simulink model "RaibertControlV2"  (R2022a)
settings: Solver=ode4  StartTime=0.0  StopTime=1  FixedStep=1/1000  RelTol=1e-3  AbsTol=1e-3  EnableMultiTasking=on
undefined symbols (not defined in the file or in its folder): Carrier, N, Ring, T, X, Y, Z
libraries: sm_lib x133, nesl_utility x25, Multibody_Parts_Lib x4, fl_lib x4
(part 6 of 8)

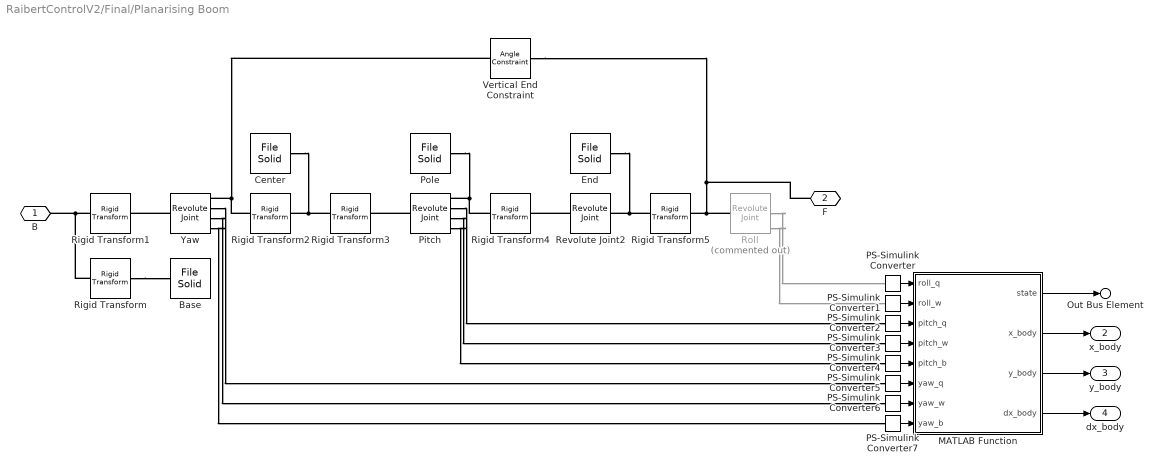
== system RaibertControlV2/Final/Planarising Boom ==
  Base : sm_lib/Body Elements/File Solid  ExtGeomFileName=meshes/boom_base.stl  UnitType=Custom  ExtGeomFileUnits=mm  StepReaderType=HEX  ExportConvexHullGeometry=off  InertiaType=Custom  Mass=16346.96  MassUnits=g  CenterOfMass=[0 10.41 0]  CenterOfMassUnits=mm  MomentsOfInertia=[161213573.39 313845541.56 161213574.63]  MomentsOfInertiaUnits=g*mm^2  ProductsOfInertia=-[32.04 0 0]  ProductsOfInertiaUnits=g*mm^2  BasedOnType=Density  Density=1000  DensityUnits=kg/m^3  DoExposeReferenceFrame=on  SerializedFrames=<Frames/>  GraphicType=FromGeometry  MarkerShape=Sphere  MarkerSize=10  GraphicVisPropType=AdvancedVisualProperties  GraphicDiffuseColor=Boom.Base.color  GraphicSpecularColor=[0.5 0.5 0.5 1.0]  GraphicAmbientColor=[0.15 0.15 0.15 1.0]  GraphicEmissiveColor=[0.0 0.0 0.0 1.0]  GraphicShininess=75  GraphicOpacity=1.0
  Center : sm_lib/Body Elements/File Solid  ExtGeomFileName=meshes/boom_center.stl  UnitType=Custom  ExtGeomFileUnits=mm  StepReaderType=HEX  ExportConvexHullGeometry=off  InertiaType=Custom  Mass=714.59  MassUnits=g  CenterOfMass=[9.30 7.66 -1.81]  CenterOfMassUnits=mm  MomentsOfInertia=[927484.76 701141.66 1377594.42]  MomentsOfInertiaUnits=g*mm^2  ProductsOfInertia=-[9906.49 -12376.64 180221.56]  ProductsOfInertiaUnits=g*mm^2  BasedOnType=Density  Density=1000  DensityUnits=kg/m^3  DoExposeReferenceFrame=on  SerializedFrames=<Frames/>  GraphicType=FromGeometry  MarkerShape=Sphere  MarkerSize=10  GraphicVisPropType=AdvancedVisualProperties  GraphicDiffuseColor=Boom.Center.color  GraphicSpecularColor=[0.5 0.5 0.5 1.0]  GraphicAmbientColor=[0.15 0.15 0.15 1.0]  GraphicEmissiveColor=[0.0 0.0 0.0 1.0]  GraphicShininess=75  GraphicOpacity=1.0
  End : sm_lib/Body Elements/File Solid  ExtGeomFileName=meshes/boom_end.stl  UnitType=Custom  ExtGeomFileUnits=mm  StepReaderType=HEX  ExportConvexHullGeometry=off  InertiaType=Custom  Mass=228  MassUnits=g  CenterOfMass=[14.63 3.02 0]  CenterOfMassUnits=mm  MomentsOfInertia=[116760.20 135814.15 68848.95]  MomentsOfInertiaUnits=g*mm^2  ProductsOfInertia=-[0 0 -1218.21]  ProductsOfInertiaUnits=g*mm^2  BasedOnType=Density  Density=1000  DensityUnits=kg/m^3  DoExposeReferenceFrame=on  SerializedFrames=<Frames/>  GraphicType=FromGeometry  MarkerShape=Sphere  MarkerSize=10  GraphicVisPropType=AdvancedVisualProperties  GraphicDiffuseColor=Boom.End.color  GraphicSpecularColor=[0.5 0.5 0.5 1.0]  GraphicAmbientColor=[0.15 0.15 0.15 1.0]  GraphicEmissiveColor=[0.0 0.0 0.0 1.0]  GraphicShininess=75  GraphicOpacity=1.0
  MATLAB Function : MATLAB Function  TreatAsAtomicUnit=on
  PS-Simulink Converter{,1..7} (8 alike) : nesl_utility/PS-Simulink Converter  PhysicalDomain=network_engine_domain  SubClassName=ps_output  LeftPortType=input  RightPortType=output  PseudoPeriodic=off  Frequencies=[]  VectorFormat=inherit  Unit=inherit  AffineConversion=off
      settings: SourceProductBaseCode=SS,PW,VE
  Pitch : sm_lib/Joints/Revolute Joint  JointMode=Normal  SenseConstraintForce=off  SenseConstraintForceX=off  SenseConstraintForceY=off  SenseConstraintForceZ=off  SenseConstraintTorque=off  SenseConstraintTorqueX=off  SenseConstraintTorqueY=off  SenseConstraintTorqueZ=off  SenseTotalForce=off  SenseTotalForceX=off  SenseTotalForceY=off  SenseTotalForceZ=off  SenseTotalTorque=off  SenseTotalTorqueX=off  SenseTotalTorqueY=off  SenseTotalTorqueZ=off  CompositeWrenchDir=FollowerOnBase  CompositeWrenchFrame=BaseFrame  EquilibriumPosition=0  EquilibriumPositionUnits=deg  SpringStiffness=0  SpringStiffnessUnits=N*m/deg  DampingCoefficient=0  DampingCoefficientUnits=N*m/(deg/s)  TorqueActuationMode=NoTorque  MotionActuationMode=ComputedMotion  SensePosition=on  SenseVelocity=on  SenseAcceleration=on  SenseTorqueForce=off  SenseLowerLimitTorqueForce=off  SenseUpperLimitTorqueForce=off  LowerLimitSpecify=off  LowerLimitBound=-90  LowerLimitBoundUnits=deg  LowerLimitStiffness=1e4  LowerLimitStiffnessUnits=N*m/deg  LowerLimitDamping=10  LowerLimitDampingUnits=N*m/(deg/s)  LowerLimitTransitionRegionWidth=0.1  LowerLimitTransitionRegionWidthUnits=deg  UpperLimitSpecify=off  UpperLimitBound=90  UpperLimitBoundUnits=deg  UpperLimitStiffness=1e4  UpperLimitStiffnessUnits=N*m/deg  UpperLimitDamping=10  UpperLimitDampingUnits=N*m/(deg/s)  UpperLimitTransitionRegionWidth=0.1  UpperLimitTransitionRegionWidthUnits=deg  PositionTargetSpecify=on  PositionTargetPriority=High  PositionTargetValue=25  PositionTargetValueUnits=deg  VelocityTargetSpecify=off  VelocityTargetPriority=High  VelocityTargetValue=10  VelocityTargetValueUnits=deg/s
  Pole : sm_lib/Body Elements/File Solid  ExtGeomFileName=meshes/boom_pole.stl  UnitType=Custom  ExtGeomFileUnits=mm  StepReaderType=HEX  ExportConvexHullGeometry=off  InertiaType=Custom  Mass=2470.66  MassUnits=g  CenterOfMass=[1149.01 0 0.46]  CenterOfMassUnits=mm  MomentsOfInertia=[1403119.37 1561987235.33 1561886539.18]  MomentsOfInertiaUnits=g*mm^2  ProductsOfInertia=-[-8.91 -1292286.42 224.67]  ProductsOfInertiaUnits=g*mm^2  BasedOnType=Density  Density=1000  DensityUnits=kg/m^3  DoExposeReferenceFrame=on  SerializedFrames=<Frames/>  GraphicType=FromGeometry  MarkerShape=Sphere  MarkerSize=10  GraphicVisPropType=AdvancedVisualProperties  GraphicDiffuseColor=Boom.Pole.color  GraphicSpecularColor=[0.5 0.5 0.5 1.0]  GraphicAmbientColor=[0.15 0.15 0.15 1.0]  GraphicEmissiveColor=[0.0 0.0 0.0 1.0]  GraphicShininess=75  GraphicOpacity=1.0
  Revolute Joint2 : sm_lib/Joints/Revolute Joint  JointMode=Normal  SenseConstraintForce=off  SenseConstraintForceX=off  SenseConstraintForceY=off  SenseConstraintForceZ=off  SenseConstraintTorque=off  SenseConstraintTorqueX=off  SenseConstraintTorqueY=off  SenseConstraintTorqueZ=off  SenseTotalForce=off  SenseTotalForceX=off  SenseTotalForceY=off  SenseTotalForceZ=off  SenseTotalTorque=off  SenseTotalTorqueX=off  SenseTotalTorqueY=off  SenseTotalTorqueZ=off  CompositeWrenchDir=FollowerOnBase  CompositeWrenchFrame=BaseFrame  EquilibriumPosition=0  EquilibriumPositionUnits=deg  SpringStiffness=0  SpringStiffnessUnits=N*m/deg  DampingCoefficient=0  DampingCoefficientUnits=N*m/(deg/s)  TorqueActuationMode=NoTorque  MotionActuationMode=ComputedMotion  SensePosition=off  SenseVelocity=off  SenseAcceleration=off  SenseTorqueForce=off  SenseLowerLimitTorqueForce=off  SenseUpperLimitTorqueForce=off  LowerLimitSpecify=off  LowerLimitBound=-90  LowerLimitBoundUnits=deg  LowerLimitStiffness=1e4  LowerLimitStiffnessUnits=N*m/deg  LowerLimitDamping=10  LowerLimitDampingUnits=N*m/(deg/s)  LowerLimitTransitionRegionWidth=0.1  LowerLimitTransitionRegionWidthUnits=deg  UpperLimitSpecify=off  UpperLimitBound=90  UpperLimitBoundUnits=deg  UpperLimitStiffness=1e4  UpperLimitStiffnessUnits=N*m/deg  UpperLimitDamping=10  UpperLimitDampingUnits=N*m/(deg/s)  UpperLimitTransitionRegionWidth=0.1  UpperLimitTransitionRegionWidthUnits=deg  PositionTargetSpecify=off  PositionTargetPriority=High  PositionTargetValue=0  PositionTargetValueUnits=deg  VelocityTargetSpecify=off  VelocityTargetPriority=High  VelocityTargetValue=0  VelocityTargetValueUnits=deg/s
  Rigid Transform : sm_lib/Frames and Transforms/Rigid Transform  TranslationMethod=None  TranslationStandardOffset=0  TranslationLengthUnit=m  TranslationStandardAxis=+Z  TranslationCartesianOffset=[0 0 0]  TranslationROffset=0  TranslationROffsetUnits=m  TranslationZOffset=0  TranslationZOffsetUnits=m  TranslationThetaOffset=0  TranslationThetaOffsetUnits=deg  RotationMethod=AlignedAxes  RotationAngleUnits=deg  RotationStandardAxis=+Z  RotationAngle=0.0  RotationArbitraryAxis=[0 0 1]  FollAlignAxisA=+Y  BaseAlignAxisA=+Z  FollAlignAxisB=+X  BaseAlignAxisB=+X  RotationSequenceAxes=FollowerAxes  RotationSequence=XYX  RotationSequenceAngles=[0 0 0]  RotationSequenceAnglesUnits=deg  RotationMatrix=[1 0 0; 0 1 0; 0 0 1]
  Rigid Transform1 : sm_lib/Frames and Transforms/Rigid Transform  TranslationMethod=StandardAxis  TranslationStandardOffset=101  TranslationLengthUnit=mm  TranslationStandardAxis=+Z  TranslationCartesianOffset=[0 0 101]  TranslationROffset=0  TranslationROffsetUnits=m  TranslationZOffset=0  TranslationZOffsetUnits=m  TranslationThetaOffset=0  TranslationThetaOffsetUnits=deg  RotationMethod=None  RotationAngleUnits=deg  RotationStandardAxis=+Z  RotationAngle=0.0  RotationArbitraryAxis=[0 0 1]  FollAlignAxisA=+Y  BaseAlignAxisA=+Z  FollAlignAxisB=+X  BaseAlignAxisB=+X  RotationSequenceAxes=FollowerAxes  RotationSequence=XYX  RotationSequenceAngles=[0 0 0]  RotationSequenceAnglesUnits=deg  RotationMatrix=[1 0 0; 0 1 0; 0 0 1]
  Rigid Transform2 : sm_lib/Frames and Transforms/Rigid Transform  TranslationMethod=None  TranslationStandardOffset=0  TranslationLengthUnit=mm  TranslationStandardAxis=+Z  TranslationCartesianOffset=[0 0 101]  TranslationROffset=0  TranslationROffsetUnits=m  TranslationZOffset=0  TranslationZOffsetUnits=m  TranslationThetaOffset=0  TranslationThetaOffsetUnits=deg  RotationMethod=AlignedAxes  RotationAngleUnits=deg  RotationStandardAxis=+Z  RotationAngle=0.0  RotationArbitraryAxis=[0 0 1]  FollAlignAxisA=+Y  BaseAlignAxisA=+Z  FollAlignAxisB=+X  BaseAlignAxisB=-X  RotationSequenceAxes=FollowerAxes  RotationSequence=XYX  RotationSequenceAngles=[0 0 0]  RotationSequenceAnglesUnits=deg  RotationMatrix=[1 0 0; 0 1 0; 0 0 1]
  Rigid Transform3 : sm_lib/Frames and Transforms/Rigid Transform  TranslationMethod=StandardAxis  TranslationStandardOffset=40  TranslationLengthUnit=mm  TranslationStandardAxis=-X  TranslationCartesianOffset=[-40 0 0]  TranslationROffset=0  TranslationROffsetUnits=m  TranslationZOffset=0  TranslationZOffsetUnits=m  TranslationThetaOffset=0  TranslationThetaOffsetUnits=deg  RotationMethod=AlignedAxes  RotationAngleUnits=deg  RotationStandardAxis=+Z  RotationAngle=0.0  RotationArbitraryAxis=[0 0 1]  FollAlignAxisA=+Y  BaseAlignAxisA=+Y  FollAlignAxisB=+X  BaseAlignAxisB=-X  RotationSequenceAxes=FollowerAxes  RotationSequence=XYX  RotationSequenceAngles=[0 0 0]  RotationSequenceAnglesUnits=deg  RotationMatrix=[1 0 0; 0 1 0; 0 0 1]
  Rigid Transform4 : sm_lib/Frames and Transforms/Rigid Transform  TranslationMethod=StandardAxis  TranslationStandardOffset=2493  TranslationLengthUnit=mm  TranslationStandardAxis=+X  TranslationCartesianOffset=[2493 0 0]  TranslationROffset=0  TranslationROffsetUnits=m  TranslationZOffset=0  TranslationZOffsetUnits=m  TranslationThetaOffset=0  TranslationThetaOffsetUnits=deg  RotationMethod=None  RotationAngleUnits=deg  RotationStandardAxis=+Z  RotationAngle=0.0  RotationArbitraryAxis=[0 0 1]  FollAlignAxisA=+Y  BaseAlignAxisA=+Y  FollAlignAxisB=+X  BaseAlignAxisB=-X  RotationSequenceAxes=FollowerAxes  RotationSequence=XYX  RotationSequenceAngles=[0 0 0]  RotationSequenceAnglesUnits=deg  RotationMatrix=[1 0 0; 0 1 0; 0 0 1]
  Rigid Transform5 : sm_lib/Frames and Transforms/Rigid Transform  TranslationMethod=StandardAxis  TranslationStandardOffset=83.5*0.62  TranslationLengthUnit=mm  TranslationStandardAxis=+X  TranslationCartesianOffset=[2493 0 0]  TranslationROffset=0  TranslationROffsetUnits=m  TranslationZOffset=0  TranslationZOffsetUnits=m  TranslationThetaOffset=0  TranslationThetaOffsetUnits=deg  RotationMethod=AlignedAxes  RotationAngleUnits=deg  RotationStandardAxis=+Z  RotationAngle=0.0  RotationArbitraryAxis=[0 0 1]  FollAlignAxisA=+Y  BaseAlignAxisA=+Y  FollAlignAxisB=+Z  BaseAlignAxisB=+X  RotationSequenceAxes=FollowerAxes  RotationSequence=XYX  RotationSequenceAngles=[0 0 0]  RotationSequenceAnglesUnits=deg  RotationMatrix=[1 0 0; 0 1 0; 0 0 1]
  Roll : sm_lib/Joints/Revolute Joint  Commented=on  JointMode=Normal  SenseConstraintForce=off  SenseConstraintForceX=off  SenseConstraintForceY=off  SenseConstraintForceZ=off  SenseConstraintTorque=off  SenseConstraintTorqueX=off  SenseConstraintTorqueY=off  SenseConstraintTorqueZ=off  SenseTotalForce=off  SenseTotalForceX=off  SenseTotalForceY=off  SenseTotalForceZ=off  SenseTotalTorque=off  SenseTotalTorqueX=off  SenseTotalTorqueY=off  SenseTotalTorqueZ=off  CompositeWrenchDir=FollowerOnBase  CompositeWrenchFrame=BaseFrame  EquilibriumPosition=0  EquilibriumPositionUnits=deg  SpringStiffness=0  SpringStiffnessUnits=N*m/deg  DampingCoefficient=0  DampingCoefficientUnits=N*m/(deg/s)  TorqueActuationMode=NoTorque  MotionActuationMode=ComputedMotion  SensePosition=on  SenseVelocity=on  SenseAcceleration=off  SenseTorqueForce=off  SenseLowerLimitTorqueForce=off  SenseUpperLimitTorqueForce=off  LowerLimitSpecify=off  LowerLimitBound=-90  LowerLimitBoundUnits=deg  LowerLimitStiffness=1e4  LowerLimitStiffnessUnits=N*m/deg  LowerLimitDamping=10  LowerLimitDampingUnits=N*m/(deg/s)  LowerLimitTransitionRegionWidth=0.1  LowerLimitTransitionRegionWidthUnits=deg  UpperLimitSpecify=off  UpperLimitBound=90  UpperLimitBoundUnits=deg  UpperLimitStiffness=1e4  UpperLimitStiffnessUnits=N*m/deg  UpperLimitDamping=10  UpperLimitDampingUnits=N*m/(deg/s)  UpperLimitTransitionRegionWidth=0.1  UpperLimitTransitionRegionWidthUnits=deg  PositionTargetSpecify=off  PositionTargetPriority=High  PositionTargetValue=0  PositionTargetValueUnits=deg  VelocityTargetSpecify=off  VelocityTargetPriority=High  VelocityTargetValue=10  VelocityTargetValueUnits=deg/s
  Vertical End Constraint : sm_lib/Constraints/Angle Constraint  ConstraintType=General  Angle=90  AngleUnits=deg  SenseSignedTorqueMagnitude=off  SenseTorque=off  SenseForce=off  WrenchDir=FollowerOnBase  WrenchFrame=BaseFrame
      settings: SourceProductBaseCode=MS
  Yaw : sm_lib/Joints/Revolute Joint  JointMode=Normal  SenseConstraintForce=off  SenseConstraintForceX=off  SenseConstraintForceY=off  SenseConstraintForceZ=off  SenseConstraintTorque=off  SenseConstraintTorqueX=off  SenseConstraintTorqueY=off  SenseConstraintTorqueZ=off  SenseTotalForce=off  SenseTotalForceX=off  SenseTotalForceY=off  SenseTotalForceZ=off  SenseTotalTorque=off  SenseTotalTorqueX=off  SenseTotalTorqueY=off  SenseTotalTorqueZ=off  CompositeWrenchDir=FollowerOnBase  CompositeWrenchFrame=BaseFrame  EquilibriumPosition=0  EquilibriumPositionUnits=deg  SpringStiffness=0  SpringStiffnessUnits=N*m/deg  DampingCoefficient=0  DampingCoefficientUnits=N*m/(deg/s)  TorqueActuationMode=NoTorque  MotionActuationMode=ComputedMotion  SensePosition=on  SenseVelocity=on  SenseAcceleration=on  SenseTorqueForce=off  SenseLowerLimitTorqueForce=off  SenseUpperLimitTorqueForce=off  LowerLimitSpecify=off  LowerLimitBound=-90  LowerLimitBoundUnits=deg  LowerLimitStiffness=1e4  LowerLimitStiffnessUnits=N*m/deg  LowerLimitDamping=10  LowerLimitDampingUnits=N*m/(deg/s)  LowerLimitTransitionRegionWidth=0.1  LowerLimitTransitionRegionWidthUnits=deg  UpperLimitSpecify=off  UpperLimitBound=90  UpperLimitBoundUnits=deg  UpperLimitStiffness=1e4  UpperLimitStiffnessUnits=N*m/deg  UpperLimitDamping=10  UpperLimitDampingUnits=N*m/(deg/s)  UpperLimitTransitionRegionWidth=0.1  UpperLimitTransitionRegionWidthUnits=deg  PositionTargetSpecify=off  PositionTargetPriority=High  PositionTargetValue=0  PositionTargetValueUnits=deg  VelocityTargetSpecify=off  VelocityTargetPriority=High  VelocityTargetValue=10  VelocityTargetValueUnits=deg/s
  B : PMIOPort  Side=Left
  F : PMIOPort  Port=2  Side=Right
  Out Bus Element : Outport  PortName=state
  x_body : Outport  Port=2
  y_body : Outport  Port=3
  dx_body : Outport  Port=4
  wires:
  PS-Simulink Converter/1 -> MATLAB Function/1(roll_q)
  PS-Simulink Converter1/1 -> MATLAB Function/2(roll_w)
  PS-Simulink Converter2/1 -> MATLAB Function/3(pitch_q)
  PS-Simulink Converter3/1 -> MATLAB Function/4(pitch_w)
  PS-Simulink Converter4/1 -> MATLAB Function/5(pitch_b)
  PS-Simulink Converter5/1 -> MATLAB Function/6(yaw_q)
  PS-Simulink Converter6/1 -> MATLAB Function/7(yaw_w)
  PS-Simulink Converter7/1 -> MATLAB Function/8(yaw_b)
  MATLAB Function/1(state) -> Out Bus Element/1
  MATLAB Function/3(y_body) -> y_body/1
  MATLAB Function/2(x_body) -> x_body/1
  MATLAB Function/4(dx_body) -> dx_body/1
  connections:
  Revolute Joint2/LConn1 -- Rigid Transform4/RConn1
  Pole/RConn1 -- Rigid Transform4/LConn1 -- Pitch/RConn1
  Center/RConn1 -- Rigid Transform3/LConn1 -- Rigid Transform2/RConn1
  Rigid Transform2/LConn1 -- Vertical End Constraint/LConn1 -- Yaw/RConn1
  End/RConn1 -- Rigid Transform5/LConn1 -- Revolute Joint2/RConn1
  Vertical End Constraint/RConn1 -- Roll/LConn1 -- Rigid Transform5/RConn1 -- F/RConn1
  Rigid Transform/RConn1 -- Base/RConn1
  Pitch/LConn1 -- Rigid Transform3/RConn1
  Rigid Transform/LConn1 -- B/RConn1 -- Rigid Transform1/LConn1
  Yaw/LConn1 -- Rigid Transform1/RConn1
  Roll/RConn2 -- PS-Simulink Converter/LConn1
  Roll/RConn3 -- PS-Simulink Converter1/LConn1
  Pitch/RConn2 -- PS-Simulink Converter2/LConn1
  Pitch/RConn3 -- PS-Simulink Converter3/LConn1
  Pitch/RConn4 -- PS-Simulink Converter4/LConn1
  Yaw/RConn2 -- PS-Simulink Converter5/LConn1
  Yaw/RConn3 -- PS-Simulink Converter6/LConn1
  Yaw/RConn4 -- PS-Simulink Converter7/LConn1

== matlab function RaibertControlV2/Final/AK90-M4/MATLAB Function ==
  data: tff_cmd input; q_cmd input; w_cmd input; Kp_cmd input; Kd_cmd input; q input; t output; w input
function t = PD(tff_cmd,q_cmd,w_cmd,Kp_cmd,Kd_cmd,q,w)
t = Kp_cmd*(q_cmd - q) + Kd_cmd*(w_cmd - w) + tff_cmd;

%function t = PD(cmd,q,w)
%t = cmd.Kp*(cmd.q - q) + cmd.Kd*(cmd.w - w) + cmd.tff;

== matlab function RaibertControlV2/Final/AK90-M3/MATLAB Function ==
  data: tff_cmd input; q_cmd input; w_cmd input; Kp_cmd input; Kd_cmd input; q input; t output; w input
function t = PD(tff_cmd,q_cmd,w_cmd,Kp_cmd,Kd_cmd,q,w)
t = Kp_cmd*(q_cmd - q) + Kd_cmd*(w_cmd - w) + tff_cmd;

%function t = PD(cmd,q,w)
%t = cmd.Kp*(cmd.q - q) + cmd.Kd*(cmd.w - w) + cmd.tff;

== matlab function RaibertControlV2/Final/Impedance Control/MATLAB Function3 ==
  data: state input; contact_offset input; stance_timer input; state output; contact_offset output; stance_timer output; t input; x_des input; x_body input; y_body input; dx_body input; foot_height output; r output; phi output; tau1 output; tau2 output; F_push input; theta1 input; theta2 input; r input; phi input; r_ref input; phi_ref input; dr input; dphi input; JT11 input; JT12 input; JT21 input; JT22 input
function [state,contact_offset,stance_timer,foot_height,r,phi,tau1,tau2]  = Controller(state,contact_offset,stance_timer,t,x_des,x_body,y_body,dx_body,F_push,theta1,theta2,r,phi,r_ref,phi_ref,dr,dphi,JT11,JT12,JT21,JT22)
%%
%     JT = [JT11,JT12;JT21,JT22];
% 
%     y_foot = r*cos(phi); % +ve value
%     % y_body --> +ve
%     % dx_body
%     
%     % constants
%     phi_neutral = phi_ref;
%     r0 = r_ref; % 0.38 0.33
%     r_min = 0.3; % 0.30 0.25
%     dt = 0.002;
%     
%     persistent state
%     persistent phi0
%     persistent contact_offset
%     persistent foot_contact
%     persistent Ts
%     persistent stance_timer
%     
%     if isempty(state)
%         state = State.Flight; %Loading
%     end
%     if isempty(phi0)
%         phi0 = phi_neutral;
%     end
%     if isempty(contact_offset)
%         contact_offset = 0;
%     end
%     if isempty(Ts)
%         Ts = 0.23; % 0.175
%     end
%     if isempty(stance_timer)
%         stance_timer = 0;
%     end
%     
%     % calculate foot contact
%     foot_height = y_body - y_foot- contact_offset; % This gets the foot height distance %- contact_offset;
%     if (foot_height > 0.005)
%         foot_contact = false;
%     else
%         foot_contact = true;
%     end
%     
%     % update stance duration
%     if foot_contact
%         stance_timer = stance_timer + dt;
%     end
%     
%     % state transitions
%     switch(state)
%     
%         case State.Flight
%             if foot_contact
%                 state = State.Loading;
%             end
%     
%         case State.Loading
%             if (dr < 0)
%                 state = State.Compression;
%             end
%     
%         case State.Compression
%             % leg velocity isn't always exactly zero
%             if ((-0.1 < dr && dr < 0.1) && (r < r_min))
%                 state = State.Thrust;
%                 contact_offset = y_body - y_foot; % update foot contact offset
%             end
%         case State.Thrust
%             if (r > r0)
%                 state = State.Unloading;
%             end
%         case State.Unloading
%             if not(foot_contact)
%                 state = State.Flight;
%                 Ts = min(stance_timer, 0.28); % record stance time
%                 stance_timer = 0; % reset stance timer
%             end
%     
%     end
%     
%     % radial thrust control
%     switch(state)
%         case State.Thrust
%             F_thrust = F_push;
%         otherwise
%             F_thrust = 0;
%     end
%     
%     % tau phi control
%     switch(state)
%         case State.Flight
%             % adjust foot placement based on horizontal velocity
%             dx_des = -min(max(1.0*(x_body - x_des), -0.5), 0.5);
%             x_foot = 0.5*dx_body*0.18 + 0.02*(dx_body - dx_des);
%             phi0 = phi_neutral + asin(x_foot / r0);
%             tau = 10*(phi0 - phi) + 1*(0 - dphi); % position foot
%         otherwise
%             tau = 0;
%     end
%     
%     
%     % permanent radial spring damper
%     Fr = 300*(r0 - r) + 15*(0 - dr) + F_thrust;
%     
%     % transform into joint torques
%     B = JT * [Fr; tau];
%     tau1 = B(1);
%     tau2 = B(2);
%     
%     %ctrl_state = state;
%%
    JT = [JT11,JT12;JT21,JT22];

    y_foot = r*cos(phi); % +ve value
    % y_body --> +ve
    % dx_body
    
    % constants
    phi_neutral = phi_ref;
    r0 = r_ref; % 0.38 0.33
    r_min = 0.33; % 0.30 0.25
    dt = 0.002;
    

    %States (1 = Flight, 2 = Loading, 3 = Compression, 4 = Thrust, 5 = Unloading)

    if t == 0
        state = 1; 
        phi0 = phi_neutral;
        contact_offset = 0;
        Ts = 0.23; % 0.175
        stance_timer = 0;
        tau1_add = 0;
        tau2_add = 0;
    end
    
    % calculate foot contact
    foot_height = y_body - y_foot %- contact_offset; % This gets the foot height distance %- contact_offset;
    if (foot_height > 0.05)
        foot_contact = false;
    else
        foot_contact = true;
    end
    
    % update stance duration
    if foot_contact
        stance_timer = stance_timer + dt;
    end
    
   % (1 = Flight, 2 = Loading, 3 = Compression, 4 = Thrust, 5 = Unloading)
    % state transitions
    if state == 1
        if foot_contact
            state = 2;
        end
    end

    if state == 2
        if (dr < 0)
            state = 3;
        end
    end

    if state == 3
        % leg velocity isn't always exactly zero
        if ((-0.2 < dr && dr < 0.2) && (r < r_min))
            state = 4;
            contact_offset = y_body - y_foot; % update foot contact offset
        end
    end
   
    if state == 4
        if (r > r0)
            state = 5;
        end
    end

    if state == 5
        if not(foot_contact)
            state = 1;
            Ts = min(stance_timer, 0.28); % record stance time
            stance_timer = 0; % reset stance timer
        end
    end
    
    
    
    if state == 4
        F_thrust = F_push;
    else
        F_thrust = 0;
    end
    
    % tau phi control

    if state == 1
        %function [tau1_add,tau2_add,knee_distance,flag] = PUSH(t,theta1,theta2)
        % End simulation if knees are too close 
        L1 = 17.5/100;
        L2 = 17.5/100;
        L5 = 12/100;
        q1 =  pi/2 - theta1; 
        q2 =  pi/2 - theta2;
        B1 = [-0.5*L5 - L1*cos(q1) ; L1*sin(q1)];
        B2 = [0.5*L5 + L2*cos(pi-q2) ; L2*sin(pi-q2)];
        knee_distance = abs(B1(1) - B2(1));
        if knee_distance<=0.08
            
            
            tau1_add = 100*0;
            tau2_add = -100*0;
            tau = 0;
        else 
            tau1_add = 0;
            tau2_add = 0;
            % adjust foot placement based on horizontal velocity
            dx_des = -min(max(1.0*(x_body - x_des), -0.5), 0.5);
            x_foot = 0.5*dx_body*0.18 + 0.02*(dx_body - dx_des);
            phi0 = phi_neutral + asin(x_foot / r0);
            tau = 10*(phi0 - phi) + 1*(0 - dphi); % position foot
        end
    else
        tau1_add = 0;
        tau2_add = 0;
        tau = 0;
    end
    
    
    % permanent radial spring damper
    Fr = 500*(r0 - r) + 25*(0 - dr) + F_thrust;
    t
    state
    foot_contact

    % transform into joint torques
    B = JT * [Fr; tau];
    tau1 = B(1) + tau1_add;
    tau2 = B(2) + tau2_add;
    
    %ctrl_state = state;
end

== matlab function RaibertControlV2/Final/Impedance Control1/MATLAB Function1 ==
  data: x_des input; foot_height output; x_body input; y_body input; dx_body input; pos1 input; vel1 input; pos2 input; vel2 input; ctrl_state output; r output; phi output; tau1 output; tau2 output
function [foot_height,ctrl_state,r,phi,tau1,tau2] = raibert_controller(x_des,x_body,y_body,dx_body,pos1,vel1,pos2,vel2) %#codegen
% calculate kinematics
[theta1,omega1,theta2,omega2] = motor2hip(pos1,vel1,pos2,vel2);
[r,phi] = fwd_polar(theta1,theta2);
[~,y_foot] = fwd_cartesian(theta1,theta2);
A = J_polar(theta1,theta2) * [omega1; omega2];
dr = A(1);
dphi = A(2);

y_foot = r*cos(phi); % +ve value
% y_body --> +ve
% dx_body

% constants
phi_neutral = 0.0;
r0 = 0.38; % 0.38 0.33
r_min = 0.3; % 0.30 0.25
dt = 0.002;

persistent state
persistent phi0
persistent contact_offset
persistent foot_contact
persistent Ts
persistent stance_timer

if isempty(state)
    state = State.Flight; %Loading
end
if isempty(phi0)
    phi0 = phi_neutral;
end
if isempty(contact_offset)
    contact_offset = 0;
end
if isempty(Ts)
    Ts = 0.23; % 0.175
end
if isempty(stance_timer)
    stance_timer = 0;
end

% calculate foot contact
foot_height = y_body - y_foot % This gets the foot height distance %- contact_offset;
if (foot_height > 0.005)
    foot_contact = false;
else
    foot_contact = true;
end

% update stance duration
if foot_contact
    stance_timer = stance_timer + dt;
end

% state transitions
switch(state)

    case State.Flight
        if foot_contact
            state = State.Loading;
        end

    case State.Loading
        if (dr < 0)
            state = State.Compression;
        end

    case State.Compression
        % leg velocity isn't always exactly zero
        if ((-0.1 < dr && dr < 0.1) && (r < r_min))
            state = State.Thrust;
            contact_offset = y_body - y_foot; % update foot contact offset
        end
    case State.Thrust
        if (r > r0)
            state = State.Unloading;
        end
    case State.Unloading
        if not(foot_contact)
            state = State.Flight;
            Ts = min(stance_timer, 0.28); % record stance time
            stance_timer = 0; % reset stance timer
        end

end

% radial thrust control
switch(state)
    case State.Thrust
        F_thrust = 50;
    otherwise
        F_thrust = 0;
end

% tau phi control
switch(state)
    case State.Flight
        % adjust foot placement based on horizontal velocity
        dx_des = -min(max(1.0*(x_body - x_des), -0.5), 0.5);
        x_foot = 0.5*dx_body*0.18 + 0.02*(dx_body - dx_des);
        phi0 = phi_neutral + asin(x_foot / r0);
        tau = 10*(phi0 - phi) + 1*(0 - dphi); % position foot
    otherwise
        tau = 0;
end


% permanent radial spring damper
Fr = 300*(r0 - r) + 15*(0 - dr) + F_thrust;

% transform into joint torques
B = transpose(J_polar(theta1,theta2)) * [Fr; tau];
tau1 = -B(1);
tau2 = -B(2);

ctrl_state = state;
end

== matlab function RaibertControlV2/Final/Impedance Control1/MATLAB Function3 ==
  data: state input; contact_offset input; stance_timer input; state output; contact_offset output; stance_timer output; t input; x_des input; x_body input; y_body input; dx_body input; foot_height output; r output; phi output; tau1 output; tau2 output; F_push input; theta1 input; theta2 input; r input; phi input; r_ref input; phi_ref input; dr input; dphi input; JT11 input; JT12 input; JT21 input; JT22 input
function [state,contact_offset,stance_timer,foot_height,r,phi,tau1,tau2]  = Controller(state,contact_offset,stance_timer,t,x_des,x_body,y_body,dx_body,F_push,theta1,theta2,r,phi,r_ref,phi_ref,dr,dphi,JT11,JT12,JT21,JT22)
%%
%     JT = [JT11,JT12;JT21,JT22];
% 
%     y_foot = r*cos(phi); % +ve value
%     % y_body --> +ve
%     % dx_body
%     
%     % constants
%     phi_neutral = phi_ref;
%     r0 = r_ref; % 0.38 0.33
%     r_min = 0.3; % 0.30 0.25
%     dt = 0.002;
%     
%     persistent state
%     persistent phi0
%     persistent contact_offset
%     persistent foot_contact
%     persistent Ts
%     persistent stance_timer
%     
%     if isempty(state)
%         state = State.Flight; %Loading
%     end
%     if isempty(phi0)
%         phi0 = phi_neutral;
%     end
%     if isempty(contact_offset)
%         contact_offset = 0;
%     end
%     if isempty(Ts)
%         Ts = 0.23; % 0.175
%     end
%     if isempty(stance_timer)
%         stance_timer = 0;
%     end
%     
%     % calculate foot contact
%     foot_height = y_body - y_foot- contact_offset; % This gets the foot height distance %- contact_offset;
%     if (foot_height > 0.005)
%         foot_contact = false;
%     else
%         foot_contact = true;
%     end
%     
%     % update stance duration
%     if foot_contact
%         stance_timer = stance_timer + dt;
%     end
%     
%     % state transitions
%     switch(state)
%     
%         case State.Flight
%             if foot_contact
%                 state = State.Loading;
%             end
%     
%         case State.Loading
%             if (dr < 0)
%                 state = State.Compression;
%             end
%     
%         case State.Compression
%             % leg velocity isn't always exactly zero
%             if ((-0.1 < dr && dr < 0.1) && (r < r_min))
%                 state = State.Thrust;
%                 contact_offset = y_body - y_foot; % update foot contact offset
%             end
%         case State.Thrust
%             if (r > r0)
%                 state = State.Unloading;
%             end
%         case State.Unloading
%             if not(foot_contact)
%                 state = State.Flight;
%                 Ts = min(stance_timer, 0.28); % record stance time
%                 stance_timer = 0; % reset stance timer
%             end
%     
%     end
%     
%     % radial thrust control
%     switch(state)
%         case State.Thrust
%             F_thrust = F_push;
%         otherwise
%             F_thrust = 0;
%     end
%     
%     % tau phi control
%     switch(state)
%         case State.Flight
%             % adjust foot placement based on horizontal velocity
%             dx_des = -min(max(1.0*(x_body - x_des), -0.5), 0.5);
%             x_foot = 0.5*dx_body*0.18 + 0.02*(dx_body - dx_des);
%             phi0 = phi_neutral + asin(x_foot / r0);
%             tau = 10*(phi0 - phi) + 1*(0 - dphi); % position foot
%         otherwise
%             tau = 0;
%     end
%     
%     
%     % permanent radial spring damper
%     Fr = 300*(r0 - r) + 15*(0 - dr) + F_thrust;
%     
%     % transform into joint torques
%     B = JT * [Fr; tau];
%     tau1 = B(1);
%     tau2 = B(2);
%     
%     %ctrl_state = state;
%%
    JT = [JT11,JT12;JT21,JT22];

    y_foot = r*cos(phi); % +ve value
    % y_body --> +ve
    % dx_body
    
    % constants
    phi_neutral = phi_ref;
    r0 = r_ref; % 0.38 0.33
    r_min = 0.33; % 0.30 0.25
    dt = 0.002;
    

    %States (1 = Flight, 2 = Loading, 3 = Compression, 4 = Thrust, 5 = Unloading)

    if t == 0
        state = 1; 
        phi0 = phi_neutral;
        contact_offset = 0;
        Ts = 0.23; % 0.175
        stance_timer = 0;
        tau1_add = 0;
        tau2_add = 0;
    end
    
    % calculate foot contact
    foot_height = y_body - y_foot %- contact_offset; % This gets the foot height distance %- contact_offset;
    if (foot_height > 0.005)
        foot_contact = false;
    else
        foot_contact = true;
    end
    
    % update stance duration
    if foot_contact
        stance_timer = stance_timer + dt;
    end
    
   % (1 = Flight, 2 = Loading, 3 = Compression, 4 = Thrust, 5 = Unloading)
    % state transitions
    if state == 1
        if foot_contact
            state = 2;
        end
    end

    if state == 2
        if (dr < 0)
            state = 3;
        end
    end

    if state == 3
        % leg velocity isn't always exactly zero
        if ((-0.1 < dr && dr < 0.1) && (r < r_min))
            state = 4;
            contact_offset = y_body - y_foot; % update foot contact offset
        end
    end
   
    if state == 4
        if (r > r0)
            state = 5;
        end
    end

    if state == 5
        if not(foot_contact)
            state = 1;
            Ts = min(stance_timer, 0.28); % record stance time
            stance_timer = 0; % reset stance timer
        end
    end
    
    
    
    if state == 4
        F_thrust = F_push;
    else
        F_thrust = 0;
    end
    
    % tau phi control

    if state == 1
        %function [tau1_add,tau2_add,knee_distance,flag] = PUSH(t,theta1,theta2)
        % End simulation if knees are too close 
        L1 = 17.5/100;
        L2 = 17.5/100;
        L5 = 12/100;
        q1 =  pi/2 - theta1; 
        q2 =  pi/2 - theta2;
        B1 = [-0.5*L5 - L1*cos(q1) ; L1*sin(q1)];
        B2 = [0.5*L5 + L2*cos(pi-q2) ; L2*sin(pi-q2)];
        knee_distance = abs(B1(1) - B2(1));
        if knee_distance<=0.08

            tau1_add = 100*0;
            tau2_add = -100*0;
            tau = 0;
        else 
            tau1_add = 0;
            tau2_add = 0;
            % adjust foot placement based on horizontal velocity
            dx_des = -min(max(1.0*(x_body - x_des), -0.5), 0.5);
            x_foot = 0.5*dx_body*0.18 + 0.02*(dx_body - dx_des);
            phi0 = (phi_neutral + asin(x_foot / r0));
            tau = 10*(phi0 - phi) + 1*(0 - dphi); % position foot
        end
    else
        tau1_add = 0;
        tau2_add = 0;
        tau = 0;
    end
    
    
    % permanent radial spring damper
    Fr = 500*(r0 - r) + 25*(0 - dr) + F_thrust;
    
    % transform into joint torques
    B = JT * [Fr; tau];
    tau1 = B(1) + tau1_add;
    tau2 = B(2) + tau2_add;
    
    %ctrl_state = state;
end

== matlab function RaibertControlV2/Final/Impedance Control/to_Polar ==
  data: theta1 input; theta2 input; r output; phi output
function [r,phi] = Position(theta1,theta2)
%POSITION
%    [R,PHI] = POSITION(THETA1,THETA2)

%    This function was generated by the Symbolic Math Toolbox version 8.6.
%    17-May-2022 09:32:07

r = sqrt((cos(acos(sqrt((sin(theta1-pi./2.0).*(7.0./4.0e+1)+sin(theta2+pi./2.0).*(7.0./4.0e+1)).^2+abs(cos(theta1-pi./2.0).*(7.0./4.0e+1)+cos(theta2+pi./2.0).*(7.0./4.0e+1)+3.0./2.5e+1).^2).*(5.0./3.0))+atan2(sin(theta1-pi./2.0).*(-7.0./4.0e+1)-sin(theta2+pi./2.0).*(7.0./4.0e+1),abs(cos(theta1-pi./2.0).*(7.0./4.0e+1)+cos(theta2+pi./2.0).*(7.0./4.0e+1)+3.0./2.5e+1))+6.012387278395987e-2).*(-3.328470665197855e-1)+cos(theta2+pi./2.0).*(7.0./4.0e+1)+3.0./5.0e+1).^2+(sin(acos(sqrt((sin(theta1-pi./2.0).*(7.0./4.0e+1)+sin(theta2+pi./2.0).*(7.0./4.0e+1)).^2+abs(cos(theta1-pi./2.0).*(7.0./4.0e+1)+cos(theta2+pi./2.0).*(7.0./4.0e+1)+3.0./2.5e+1).^2).*(5.0./3.0))+atan2(sin(theta1-pi./2.0).*(-7.0./4.0e+1)-sin(theta2+pi./2.0).*(7.0./4.0e+1),abs(cos(theta1-pi./2.0).*(7.0./4.0e+1)+cos(theta2+pi./2.0).*(7.0./4.0e+1)+3.0./2.5e+1))+6.012387278395987e-2).*3.328470665197855e-1+sin(theta2+pi./2.0).*(7.0./4.0e+1)).^2);
if nargout > 1
    phi = pi./2.0-angle(cos(acos(sqrt((sin(theta1-pi./2.0).*(7.0./4.0e+1)+sin(theta2+pi./2.0).*(7.0./4.0e+1)).^2+abs(cos(theta1-pi./2.0).*(7.0./4.0e+1)+cos(theta2+pi./2.0).*(7.0./4.0e+1)+3.0./2.5e+1).^2).*(5.0./3.0))+atan2(sin(theta1-pi./2.0).*(-7.0./4.0e+1)-sin(theta2+pi./2.0).*(7.0./4.0e+1),abs(cos(theta1-pi./2.0).*(7.0./4.0e+1)+cos(theta2+pi./2.0).*(7.0./4.0e+1)+3.0./2.5e+1))+6.012387278395987e-2).*(-3.328470665197855e-1)+sin(acos(sqrt((sin(theta1-pi./2.0).*(7.0./4.0e+1)+sin(theta2+pi./2.0).*(7.0./4.0e+1)).^2+abs(cos(theta1-pi./2.0).*(7.0./4.0e+1)+cos(theta2+pi./2.0).*(7.0./4.0e+1)+3.0./2.5e+1).^2).*(5.0./3.0))+atan2(sin(theta1-pi./2.0).*(-7.0./4.0e+1)-sin(theta2+pi./2.0).*(7.0./4.0e+1),abs(cos(theta1-pi./2.0).*(7.0./4.0e+1)+cos(theta2+pi./2.0).*(7.0./4.0e+1)+3.0./2.5e+1))+6.012387278395987e-2).*3.328470665197855e-1i+cos(theta2+pi./2.0).*(7.0./4.0e+1)+sin(theta2+pi./2.0).*1.75e-1i+3.0./5.0e+1);
end
